simulink model "demowpt"  (Simulink 6.1)
settings: Solver=ode45  StartTime=0.0  StopTime=50  MaxStep=10^-2  RelTol=1e-3
libraries: simulink x3, Marine_GNC x1
settings Model: LastModifiedBy=perez
settings DataIOCC: SignalLoggingName=sigsOut
settings OptimizationCC: BooleanDataType=off  InlineInvariantSignals=off
settings HardwareCC: TargetUnknown=on
settings CodeAppCC: IgnoreCustomStorageClasses=off
settings STFCustomTargetCC: TargetFcnLib=ansi_tfl_tmw.mat  GenFloatMathFcnCalls=ANSI_C  ModelReferenceCompliant=off  SystemTargetFile=grt.tlc

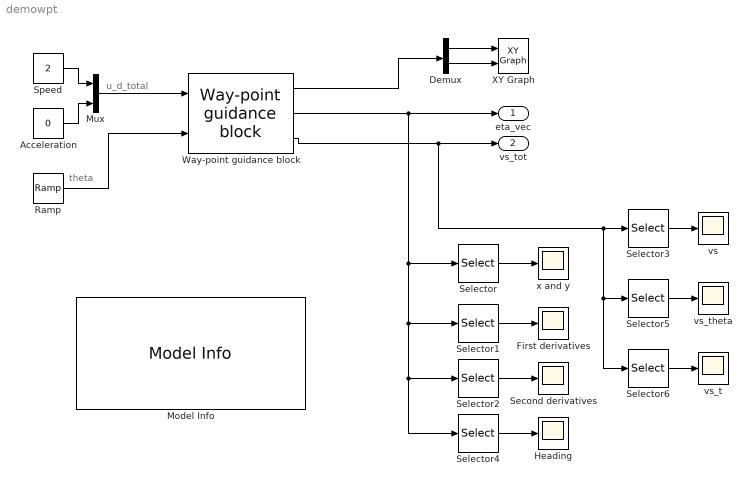
== system demowpt ==
  note: u_d_total
  note: theta
  Acceleration : Constant  Value=0
  Demux : Demux  Outputs=2
  First derivatives : Scope
      settings: TimeRange=14  YMin=-2000  YMax=2500
  Heading : Scope
      settings: TimeRange=14  YMin=-4  YMax=4  SaveName=ScopeData3
  Model Info : simulink/Model-Wide Utilities/Model Info  InitialBlockCM=None  BlockCM=None  Frame=on  DisplayStringWithTags=|  HorizontalTextAlignment=Left  LeftAlignmentValue=0.02  SourceBlockDiagram=demowpt  TagMaxNumber=20
      | Way-point Guidance Demo.
      | Creates a 3 times differentiable path between 
      | the provided way-points. The user can choose
      | between cubic splines (3rd order)  and a 5th
      | order polynomial.
      | Author: Jørgen Corneliussen
      | %<ModifiedDate>
  Mux : Mux  Inputs=2
  Ramp : simulink/Sources/Ramp  slope=1  start=0  X0=0
  Second derivatives : Scope
      settings: TimeRange=14  YMin=-8000  YMax=8000  SaveName=ScopeData5
  Selector : Selector  Elements=[1 2]  InputPortWidth=9
  Selector1 : Selector  Elements=[4 5]  InputPortWidth=9
  Selector2 : Selector  Elements=[7 8]  InputPortWidth=9
  Selector3 : Selector  InputPortWidth=3
  Selector4 : Selector  Elements=3  InputPortWidth=9
  Selector5 : Selector  Elements=2  InputPortWidth=3
  Selector6 : Selector  Elements=3  InputPortWidth=3
  Speed : Constant  Value=2
  Way-point guidance block : Marine_GNC/Guidance/Way-point guidance block  x_vector=[-800 -500 -200 -50 -200 -250 200 500 500 300 0 -300 -600]  y_vector=[100 1800 2000 1500 1000 100 1000 300 -250 -200 100 -600 -1000]  method=5th order polynomial  drawmode=on  stop=on  mode=Acc  start=[100 0]  final=[0 100]  constraint=off
  XY Graph : simulink/Sinks/XY Graph  xmin=-800  xmax=600  ymin=-1500  ymax=2500  st=-1
  vs : Scope
      settings: TimeRange=4.5  YMin=-0.00788177  YMax=0.0507389
  vs_t : Scope
      settings: TimeRange=10  SaveName=ScopeData6
  vs_theta : Scope
      settings: TimeRange=14  YMin=-50000  YMax=450000  SaveName=ScopeData4
  x and y : Scope
      settings: TimeRange=14  YMin=-1000  YMax=2500  SaveName=ScopeData2
  eta_vec : Outport
  vs_tot : Outport  Port=2
  wires:
  Speed/1 -> Mux/1
  Acceleration/1 -> Mux/2
  Mux/1 -> Way-point guidance block/1
  Way-point guidance block/2 -> eta_vec/1, Selector/1, Selector1/1, Selector2/1, Selector4/1
  Ramp/1 -> Way-point guidance block/2
  Way-point guidance block/3 -> vs_tot/1, Selector3/1, Selector6/1, Selector5/1
  Selector/1 -> x and y/1
  Selector1/1 -> First derivatives/1
  Selector2/1 -> Second derivatives/1
  Way-point guidance block/1 -> Demux/1
  Selector3/1 -> vs/1
  Selector4/1 -> Heading/1
  Selector5/1 -> vs_theta/1
  Selector6/1 -> vs_t/1
  Demux/1 -> XY Graph/1
  Demux/2 -> XY Graph/2
